simulink library "tqd"  (R2021b)
settings: Solver=VariableStepAuto  StartTime=0.0  StopTime=10.0  RelTol=1e-3
undefined symbols (not defined in the file or in its folder): ATQD_APSDecReq_X_kph, ATQD_APSDecReq_Y_mps2, ATQD_APSDecReqCMD_X_kph, ATQD_APSDecReqTs_X_pct, ATQD_APSDecTimeGain_X_Deg, ATQD_APSDecTimeGain_Y_s, ATQD_APSReqLowSpd_X_Deg, ATQD_AutoHoldReleaseBPS_X_Deg, ATQD_AWDLoadTrqnsGain_X_kg, ATQD_AWDLoadTrqnsGain_Y_pct, ATQD_BOSEnBPSPosn_X_kph, ATQD_BOSMap_X_rpm, ATQD_BOSMap_Y_pct, ATQD_CreepBaseTqD_X_kph, ATQD_CreepBaseTqD_Y_Deg, ATQD_CreepBaseTqR_X_kph, ATQD_CreepBaseTqR_Y_Deg, ATQD_CreepBPSDisPosn_X_Deg, ATQD_CreepBPSDisPosnR_X_Deg, ATQD_CreepBPSEnPosn_X_Deg, ATQD_CreepBPSEnPosnR_X_Deg, ATQD_CreepDeltaTq_X_kph, ATQD_CreepIterm_X_kph, ATQD_CreepIterm_Y_kph, ATQD_CreepItermMaxLimit_X_pct, ATQD_CreepPreloadTime_X_kph, ATQD_CreepPreloadTq_X_kph, ATQD_CreepPreloadTq_Y_s, ATQD_CreepProtTq_X_Deg, ATQD_CreepPterm_X_kph, ATQD_ECOTqMapD_X_rpm, ATQD_ECOTqMapD_Y_pct, ATQD_EOPDTqMapDCon_X_rpm, ATQD_EOPDTqMapDCon_Y_Deg, ATQD_EstInitVehWeight_X_c, ATQD_LHMRollGenMapD_X_rpm, ATQD_LHMRollGenMapD_Y_rpm, ATQD_LHMTqMapD_X_rpm, ATQD_LHMTqMapD_Y_pct, ATQD_NL1TqMapD_X_rpm, ATQD_NL1TqMapD_Y_pct, ATQD_NOPDTqMapDCon_X_rpm, ATQD_NOPDTqMapDCon_Y_Deg, ATQD_NRMRrEDUSpRat_X_rpm, ATQD_NRMRrEDUSpRat_Y_Nm, ATQD_OPDHoldDownRelDelay_X_Deg, ATQD_OPDHoldEnSpd_X_Deg, ATQD_OPDHoldRelDetTime_X_Deg, ATQD_OPDHoldReleaseTq_X_Deg, ATQD_OrigPedTqLowLim_X_Deg, ATQD_OrigPedTqLowLim_Y_pct, ATQD_PedalMapClimbUpLim_X_rpm, ATQD_PedalMapClimbUpLim_Y_Deg, ATQD_PreLoadTq_X_s, ATQD_RollGenMapEL1_X_rpm, ATQD_RollGenMapEL1_Y_rpm, ATQD_SL1TqMapD_X_rpm, ATQD_SL1TqMapD_Y_pct, ATQD_SlideRegenTqGain_X_Gps, ATQD_SlideRegenTqGain_Y_pct ... (+444)
libraries: hcu_lib x70, simulink x61, tqr x1
(part 11 of 14)

== system tqd/TQD/TorqueDemand/TorqueModule/OPD Hold/Release Condition ==
  VVMC_EstSlope_Deg : Inport
  VTQD_VehActSpd_kph : Inport  Port=2
  VTQR_NoABSFEDUWhlTqReq_Nm : Inport  Port=3
  VTQR_NoABSREDUWhlTqReq_Nm : Inport  Port=4
  VTQD_ActBPSPosn_pct : Inport  Port=5
  task_time_s : Inport  Port=6
  VTQD_APSReqTimer_s : Inport  Port=7
  VTQD_LowIdleAccPedal_flg : Inport  Port=8
  VTQD_OPDHoldRgnOn2Off_flg : Inport  Port=9
  VTQD_ActAPSPosn_pct : Inport  Port=10
  VTQD_FrOPDHoldRelTqGain_Nm : Inport  Port=11
  VTQD_RrOPDHoldRelTqGain_Nm : Inport  Port=12
  AND : Logic  Inputs=3  AllPortsSameDT=off  OutDataTypeStr=boolean
  AND1 : Logic  AllPortsSameDT=off  OutDataTypeStr=boolean
  AND2 : Logic  AllPortsSameDT=off  OutDataTypeStr=boolean
  AND3 : Logic  AllPortsSameDT=off  OutDataTypeStr=boolean
  Add : Sum
  Add1 : Sum  Inputs=+-+
  Add6 : Sum
  Add7 : Sum
  Constant1 : Constant  Value=KTQD_APSRelDisTqDev_Nm
  Constant{5,10,23,30} (4 alike) : Constant  Value=ZERO_FLOAT
  Constant2 : Constant  Value=KTQD_OPDHoldDownEnTime_s
  Constant36 : Constant  Value=KTQD_OPDHoldRelDetSpd_kph
  Constant4 : Constant  Value=KTQD_OPDHoldRelTqGain_Nm
  Constant6 : Constant  Value=KTQD_OPDHoldDetRevSpd_kph
  Constant7 : Constant  Value=KTQD_OPDHoldLiftRevSpd_kph
  Constant8 : Constant  Value=KTQD_APSDecReqMaxTime_s
  Constant9 : Constant  Value=KTQD_OPDHoldRelTqGain_Nm
  Delay{,1..3} (4 alike) : Delay  DelayLength=1
  DelayEnable : hcu_lib/Basic_Blocks/DelayEnable
  DelayEnable1 : hcu_lib/Basic_Blocks/DelayEnable
  Detect Increase : simulink/Logic and Bit Operations/Detect Increase  vinit=0.0  OutDataTypeStr=boolean
  Detect Increase1 : simulink/Logic and Bit Operations/Detect Increase  vinit=0.0  OutDataTypeStr=boolean
  Detect Increase2 : simulink/Logic and Bit Operations/Detect Increase  vinit=0.0  OutDataTypeStr=boolean
  MTQD_AutoHoldReleaseBPS_Y_pct : Lookup_n-D  NumberOfTableDimensions=1  BreakpointsForDimension1=ATQD_AutoHoldReleaseBPS_X_Deg  Table=MTQD_AutoHoldReleaseBPS_Y_pct  InternalRulePriority=Speed  RndMeth=Simplest  InputSameDT=on
  MTQD_OPDHoldDownRelDelay_Y_s : Lookup_n-D  NumberOfTableDimensions=1  BreakpointsForDimension1=ATQD_OPDHoldDownRelDelay_X_Deg  Table=MTQD_OPDHoldDownRelDelay_Y_s  InternalRulePriority=Speed  RndMeth=Simplest  InputSameDT=on
  MTQD_OPDHoldRelDetTime_Y_s : Lookup_n-D  NumberOfTableDimensions=1  BreakpointsForDimension1=ATQD_OPDHoldRelDetTime_X_Deg  Table=MTQD_OPDHoldRelDetTime_Y_s  InternalRulePriority=Speed  RndMeth=Simplest  InputSameDT=on
  MTQD_OPDHoldReleaseTq_Y_Nm{,1..3} (4 alike) : Lookup_n-D  NumberOfTableDimensions=1  BreakpointsForDimension1=ATQD_OPDHoldReleaseTq_X_Deg  Table=MTQD_OPDHoldReleaseTq_Y_Nm  InternalRulePriority=Speed  RndMeth=Simplest  InputSameDT=on
  Max : MinMax  Function=max  Inputs=2
  Max1 : MinMax  Function=max  Inputs=2
  Max2 : MinMax  Function=max  Inputs=2
  NOT{,1..5} (6 alike) : Logic  Operator=NOT  AllPortsSameDT=off  OutDataTypeStr=boolean
  OR : Logic  Operator=OR  AllPortsSameDT=off  OutDataTypeStr=boolean
  OR1 : Logic  Operator=OR  AllPortsSameDT=off  OutDataTypeStr=boolean
  OR2 : Logic  Operator=OR  AllPortsSameDT=off  OutDataTypeStr=boolean
  OR3 : Logic  Operator=OR  Inputs=3  AllPortsSameDT=off  OutDataTypeStr=boolean
  Relational Operator : RelationalOperator  Operator=>  OutDataTypeStr=boolean  RndMeth=Simplest
  Relational Operator1 : RelationalOperator  Operator=<=  OutDataTypeStr=boolean  RndMeth=Simplest
  Relational Operator3 : RelationalOperator  Operator=<=  OutDataTypeStr=boolean  RndMeth=Simplest
  Relational Operator4 : RelationalOperator  OutDataTypeStr=boolean  RndMeth=Simplest
  Relational Operator5 : RelationalOperator  Operator=<  OutDataTypeStr=boolean  RndMeth=Simplest
  Relational Operator6 : RelationalOperator  Operator=>  OutDataTypeStr=boolean  RndMeth=Simplest
  Relational Operator7 : RelationalOperator  OutDataTypeStr=boolean  RndMeth=Simplest
  Relational Operator9 : RelationalOperator  OutDataTypeStr=boolean  RndMeth=Simplest
  Relay : Relay  OnSwitchValue=KTQD_OPDHoldGradeUp_Deg  OffSwitchValue=KTQD_OPDHoldGradeDown_Deg  OutDataTypeStr=boolean
  Relay1 : Relay  OnSwitchValue=KTQD_OPDHoldGradeUp_Deg  OffSwitchValue=KTQD_OPDHoldGradeDown_Deg  OutDataTypeStr=boolean
  SR_Latch : hcu_lib/Basic_Blocks/SR_Latch
  SR_Latch1 : hcu_lib/Basic_Blocks/SR_Latch
  Switch{,1..6} (7 alike) : Switch  Criteria=u2 > Threshold
  Terminator : Terminator
  VTQD_AutoHoldRelease_flg : Outport
  VTQD_OPDHoldEnRel_flg : Outport  Port=2
  VTQD_OPDHoldActRelTq_Nm : Outport  Port=3
  wires:
  VVMC_EstSlope_Deg/1 -> [VVMC_EstSlope_Deg]
  VTQD_VehActSpd_kph/1 -> [VTQD_VehActSpd_kph]
  VTQR_NoABSFEDUWhlTqReq_Nm/1 -> [VTQR_NoABSFEDUWhlTqReq_Nm]
  VTQR_NoABSREDUWhlTqReq_Nm/1 -> [VTQR_NoABSREDUWhlTqReq_Nm]
  VTQD_ActBPSPosn_pct/1 -> [VTQD_ActBPSPosn_pct]
  task_time_s/1 -> [task_time_s]
  [VTQD_AutoHoldRelease_flg] -> VTQD_AutoHoldRelease_flg/1
  [VTQD_OPDHoldEnRel_flg] -> VTQD_OPDHoldEnRel_flg/1
  VTQD_APSReqTimer_s/1 -> [VTQD_APSReqTimer_s]
  VTQD_LowIdleAccPedal_flg/1 -> [VTQD_LowIdleAccPedal_flg]
  VTQD_OPDHoldRgnOn2Off_flg/1 -> [VTQD_OPDHoldRgnOn2Off_flg]
  VTQD_ActAPSPosn_pct/1 -> Terminator/1
  VTQD_RrOPDHoldRelTqGain_Nm/1 -> [VTQD_RrOPDHoldRelTqGain_Nm]
  VTQD_FrOPDHoldRelTqGain_Nm/1 -> [VTQD_FrOPDHoldRelTqGain_Nm]
  SR_Latch/1 -> DelayEnable/1  "VTQD_OPDHoldEnRelLatch_flg"
  Detect Increase2/1 -> OR2/1
  Detect Increase1/1 -> SR_Latch1/1
  DelayEnable1/1 -> Switch1/1
  SR_Latch1/1 -> [VTQD_OPDHoldRelReverse_flg]  "VTQD_OPDHoldRelReverse_flg"
  MTQD_OPDHoldDownRelDelay_Y_s/1 -> [VTQD_OPDHoldDownRelDelay_s]  "VTQD_OPDHoldDownRelDelay_s"
  Constant4/1 -> Switch2/1
  [VVMC_EstSlope_Deg] -> MTQD_OPDHoldDownRelDelay_Y_s/1
  [task_time_s] -> DelayEnable1/3
  [VTQD_LowIdleAccPedal_flg] -> NOT2/1
  Constant30/1 -> Switch5/1
  NOT/1 -> AND/2
  [VVMC_EstSlope_Deg] -> Relay1/1
  Relay1/1 -> NOT3/1
  Constant2/1 -> Relational Operator1/2
  OR1/1 -> AND/3
  Switch1/1 -> Switch/3
  AND2/1 -> Switch1/3
  [VTQD_LowIdleAccPedal_flg] -> NOT1/1
  [VTQD_OPDHoldRgnOn2Off_flg] -> Switch/2
  Relational Operator/1 -> OR1/1
  Relational Operator1/1 -> AND/1
  [VTQD_OPDHoldRelDetTime_s] -> DelayEnable/2
  AND/1 -> OR/1
  [VVMC_EstSlope_Deg] -> Relay/1
  [VTQR_NoABSFEDUWhlTqReq_Nm] -> Add6/1
  [VTQR_NoABSREDUWhlTqReq_Nm] -> Add6/2
  [task_time_s] -> DelayEnable/3
  [VTQR_NoABSFEDUWhlTqReq_Nm] -> Add7/1
  [VTQD_ActBPSPosn_pct] -> Relational Operator/1
  Add1/1 -> Max1/1
  [VVMC_EstSlope_Deg] -> MTQD_OPDHoldReleaseTq_Y_Nm/1
  DelayEnable/1 -> [VTQD_OPDHoldEnRel_flg]  "VTQD_OPDHoldEnRel_flg"
  [VTQR_NoABSREDUWhlTqReq_Nm] -> Add7/2
  Max1/1 -> Relational Operator5/2
  [VTQD_VehActSpd_kph] -> Relational Operator9/1
  Relational Operator9/1 -> Switch5/2
  [VVMC_EstSlope_Deg] -> MTQD_AutoHoldReleaseBPS_Y_pct/1
  [VVMC_EstSlope_Deg] -> MTQD_OPDHoldRelDetTime_Y_s/1
  Switch5/1 -> [VTQD_OPDHoldRelDetTime_s]  "VTQD_OPDHoldRelDetTime_s"
  MTQD_AutoHoldReleaseBPS_Y_pct/1 -> Relational Operator/2  "VTQD_AutoHoldReleaseAPS_pct"
  OR/1 -> [VTQD_AutoHoldRelease_flg]  "VTQD_AutoHoldRelease_flg"
  MTQD_OPDHoldReleaseTq_Y_Nm/1 -> Switch6/3
  Relational Operator3/1 -> Detect Increase1/1
  [VTQD_OPDHoldDownRelDelay_s] -> DelayEnable1/2
  Delay3/1 -> Max2/1
  Max2/1 -> Switch6/1
  Constant6/1 -> Relational Operator3/2
  Detect Increase/1 -> OR3/1
  Add7/1 -> Relational Operator5/1  "VTQD_OPDHoldDisRelTq_Nm"
  Switch6/1 -> Add/2, Delay3/1  "VTQD_OPDHoldReleaseTq_Nm"
  [VVMC_EstSlope_Deg] -> MTQD_OPDHoldReleaseTq_Y_Nm3/1
  [VTQD_APSReqTimer_s] -> Delay/1
  NOT3/1 -> Switch1/2
  [VTQD_OPDHoldRelReverse_flg] -> Detect Increase2/1
  [VTQD_OPDHoldRelReverse_flg] -> Switch6/2
  Constant23/1 -> Max1/2
  [VTQD_LowIdleAccPedal_flg] -> NOT4/1
  MTQD_OPDHoldRelDetTime_Y_s/1 -> Switch5/3
  [VTQD_OPDHoldRelReverse_flg] -> Switch3/2
  Relational Operator4/1 -> SR_Latch/1  "VTQD_OPDHoldEnRelease_flg"
  Switch2/1 -> Add/1
  NOT5/1 -> AND2/2
  MTQD_OPDHoldReleaseTq_Y_Nm1/1 -> Switch4/3
  Relay/1 -> NOT/1
  Add/1 -> [VTQD_OPDHoldActRelTq_Nm], Relational Operator4/2  "VTQD_OPDHoldActRelTq_Nm"
  [VTQD_OPDHoldRelReverse_flg] -> Switch4/2
  Delay/1 -> Relational Operator1/1
  Constant8/1 -> Relational Operator7/2
  OR2/1 -> SR_Latch/2
  [VTQD_VehActSpd_kph] -> Relational Operator3/1
  Delay2/1 -> Max/1
  [VTQD_OPDHoldEnRel_flg] -> AND1/2
  AND1/1 -> Switch/1
  [VTQD_LowIdleAccPedal_flg] -> AND3/1
  [VTQD_LowIdleAccPedal_flg] -> NOT5/1
  Constant36/1 -> Relational Operator9/2
  NOT4/1 -> DelayEnable1/1
  [VTQD_APSReqTimer_s] -> Delay1/1
  Constant10/1 -> Switch3/3
  MTQD_OPDHoldReleaseTq_Y_Nm2/1 -> Max/2
  [VTQD_LowIdleAccPedal_flg] -> Detect Increase/1
  Add6/1 -> Relational Operator4/1  "VTQD_OPDHoldEnRelTq_flg"
  [VTQD_OPDHoldRelReverse_flg] -> Switch2/2
  Switch3/1 -> Add1/1
  [VVMC_EstSlope_Deg] -> MTQD_OPDHoldReleaseTq_Y_Nm1/1
  Relational Operator5/1 -> OR2/2  "VTQD_OPDHoldDisRelease_flg"
  MTQD_OPDHoldReleaseTq_Y_Nm3/1 -> Max2/2
  Delay1/1 -> Relational Operator7/1
  Relational Operator7/1 -> AND3/2
  Constant7/1 -> Relational Operator6/2
  Switch4/1 -> Delay2/1, Add1/3
  Constant5/1 -> Switch2/3
  AND3/1 -> OR3/3
  Constant9/1 -> Switch3/1
  Switch/1 -> OR/2
  NOT2/1 -> AND1/1
  [VTQD_VehActSpd_kph] -> Relational Operator6/1
  [VTQD_OPDHoldEnRel_flg] -> AND2/1
  Constant1/1 -> Add1/2
  NOT1/1 -> OR1/2
  Relational Operator6/1 -> OR3/2
  Max/1 -> Switch4/1
  [VVMC_EstSlope_Deg] -> MTQD_OPDHoldReleaseTq_Y_Nm2/1
  OR3/1 -> SR_Latch1/2
  [VTQD_OPDHoldActRelTq_Nm] -> VTQD_OPDHoldActRelTq_Nm/1

== system tqd/TQD/TorqueDemand/TorqueModule/OPD Hold/System Status ==
  VTQD_GearActualPosn_enum : Inport
  VINP_EPBSta_enum : Inport  Port=2
  VTQD_RegenMode_enum : Inport  Port=3
  VTQD_AutiHoldRelease_flg : Inport  Port=4
  VTQD_AntiBlockRrActDisTime_s : Inport  Port=5
  VTQD_RrAntiBlockAactive_flg : Inport  Port=6
  VTQD_ActBPSPosn_pct : Inport  Port=7
  VTQD_AntiBlockFrActDisTime_s : Inport  Port=8
  VTQD_FrAntiBlockAactive_flg : Inport  Port=9
  VVMC_ADASActive_flg : Inport  Port=10
  VPMM_PwrSta_enum : Inport  Port=11
  VVMC_CruzActive_flg : Inport  Port=12
  VTQD_VehActSpd_kph : Inport  Port=13
  AND2 : Logic  Inputs=6  AllPortsSameDT=off  OutDataTypeStr=boolean
  AND5 : Logic  AllPortsSameDT=off  OutDataTypeStr=boolean
  AND6 : Logic  AllPortsSameDT=off  OutDataTypeStr=boolean
  Constant1 : Constant  Value=2  OutDataTypeStr=uint8
  Constant2 : Constant  Value=0  OutDataTypeStr=uint8
  Constant3 : Constant  Value=ENUM_EPBSTA_APPLIED
  Constant4 : Constant  Value=ENUM_GEARACTUALPOSN_P
  Constant40 : Constant  Value=ENUM_REGENLEVEL_OPD
  Constant44 : Constant  Value=ENUM_REGENLEVEL_OPD
  Constant45 : Constant  Value=ENUM_POWERSTA_READY
  Constant5 : Constant  Value=ENUM_GEARACTUALPOSN_D
  Constant6 : Constant  Value=KTQD_AutoHoldEnSpd_kph
  Constant7 : Constant  Value=ENUM_EPBSTA_APPLIED
  Delay : Delay  DelayLength=1
  Equal{1..2,8,11,30} (5 alike) : RelationalOperator  Operator===  OutDataTypeStr=boolean  RndMeth=Simplest
  Equal10 : RelationalOperator  Operator=~=  OutDataTypeStr=boolean  RndMeth=Simplest
  Equal3 : RelationalOperator  Operator=~=  OutDataTypeStr=boolean  RndMeth=Simplest
  GreaterThan3 : RelationalOperator  Operator=>  OutDataTypeStr=boolean  RndMeth=Simplest
  NOT3 : Logic  Operator=NOT  AllPortsSameDT=off  OutDataTypeStr=boolean
  NOT4 : Logic  Operator=NOT  AllPortsSameDT=off  OutDataTypeStr=boolean
  OR1 : Logic  Operator=OR  AllPortsSameDT=off  OutDataTypeStr=boolean
  OR5 : Logic  Operator=OR  AllPortsSameDT=off  OutDataTypeStr=boolean
  Relational Operator3 : RelationalOperator  Operator=<=  OutDataTypeStr=boolean  RndMeth=Simplest
  SR_Latch3 : hcu_lib/Basic_Blocks/SR_Latch
  Switch : Switch  Criteria=u2 > Threshold
  Unit Delay1 : UnitDelay  SampleTime=-1  HasFrameUpgradeWarning=on
  VTQD_APSStaSys_enum : Outport
  VTQD_OPDHoldDelayForP_flg : Outport  Port=2
  VTQD_OPDHoldRgnOn2Off_flg : Outport  Port=3
  wires:
  Constant6/1 -> Relational Operator3/2
  [VVMC_CruzActive_flg] -> NOT4/1
  NOT4/1 -> AND2/4
  Relational Operator3/1 -> AND2/5
  OR1/1 -> AND2/3
  Switch/1 -> [VTQD_APSStaSys_enum]  "VTQD_APSStaSys_enum"
  [VTQD_VehActSpd_kph] -> Relational Operator3/1
  Equal2/1 -> OR1/1
  Constant2/1 -> Switch/3
  AND2/1 -> Switch/2
  Constant1/1 -> Switch/1
  [VTQD_GearActualPosn_enum] -> Equal2/1
  [VTQD_GearActualPosn_enum] -> Equal1/1
  Equal1/1 -> AND5/1
  AND5/1 -> [VTQD_OPDHoldDelayForP_flg]  "VTQD_OPDHoldDelayForP_flg"
  Equal10/1 -> AND5/2
  [VTQD_RegenMode_enum] -> Equal8/1
  OR5/1 -> [VTQD_AntiBlockEnOPDHold_flg]  "VTQD_AntiBlockEnOPDHold_flg"
  Equal8/1 -> OR5/2
  Constant40/1 -> Equal8/2
  Equal11/1 -> GreaterThan3/2, Unit Delay1/1
  SR_Latch3/1 -> [VTQD_OPDHoldRgnOn2Off_flg]  "VTQD_OPDHoldRgnOn2Off_flg"
  GreaterThan3/1 -> AND6/2
  Constant45/1 -> Equal30/2
  AND6/1 -> SR_Latch3/1
  [VPMM_PwrSta_enum] -> Equal30/1
  Equal30/1 -> AND6/1
  Unit Delay1/1 -> GreaterThan3/1
  [VTQD_AutiHoldRelease_flg] -> Delay/1
  Constant44/1 -> Equal11/2
  [VTQD_RegenMode_enum] -> Equal11/1
  Constant3/1 -> Equal10/2
  [VINP_EPBSta_enum] -> Equal10/1
  Constant4/1 -> Equal1/2
  Constant5/1 -> Equal2/2
  [VVMC_ADASActive_flg] -> NOT3/1
  NOT3/1 -> AND2/1
  [VTQD_AntiBlockEnOPDHold_flg] -> AND2/2
  [VTQD_OPDHoldRgnOn2Off_flg] -> OR5/1
  VTQD_GearActualPosn_enum/1 -> [VTQD_GearActualPosn_enum]
  VINP_EPBSta_enum/1 -> [VINP_EPBSta_enum]
  VTQD_RegenMode_enum/1 -> [VTQD_RegenMode_enum]
  VTQD_AutiHoldRelease_flg/1 -> [VTQD_AutiHoldRelease_flg]
  VTQD_AntiBlockRrActDisTime_s/1 -> [VTQD_AntiBlockRrActDisTime_s]
  VTQD_RrAntiBlockAactive_flg/1 -> [VTQD_RrAntiBlockAactive_flg]
  VTQD_ActBPSPosn_pct/1 -> [VTQD_ActBPSPosn_pct]
  VTQD_AntiBlockFrActDisTime_s/1 -> [VTQD_AntiBlockFrActDisTime_s]
  VTQD_FrAntiBlockAactive_flg/1 -> [VTQD_FrAntiBlockAactive_flg]
  VVMC_ADASActive_flg/1 -> [VVMC_ADASActive_flg]
  VPMM_PwrSta_enum/1 -> [VPMM_PwrSta_enum]
  [VTQD_OPDHoldDelayForP_flg] -> OR1/2
  VVMC_CruzActive_flg/1 -> [VVMC_CruzActive_flg]
  VTQD_VehActSpd_kph/1 -> [VTQD_VehActSpd_kph]
  [VTQD_APSStaSys_enum] -> VTQD_APSStaSys_enum/1
  [VTQD_OPDHoldDelayForP_flg] -> VTQD_OPDHoldDelayForP_flg/1
  [VTQD_OPDHoldRgnOn2Off_flg] -> VTQD_OPDHoldRgnOn2Off_flg/1
  Constant7/1 -> Equal3/2
  [VINP_EPBSta_enum] -> Equal3/1
  Equal3/1 -> AND2/6
  Delay/1 -> SR_Latch3/2

== system tqd/TQD/TorqueDemand/TorqueModule/TqCoordination/Coordinate_ADAS ==
  VVMC_ADASWhlTqReq_Nm : Inport
  VTQD_PreLoadHold_flg : Inport  Port=2
  VTQD_DriverWhlTqDem_Nm : Inport  Port=3
  Action Port : ActionPort
  Constant9 : Constant  Value=ENUM_TQSOURCE_ADAS
  Switch : Switch  Criteria=u2 > Threshold
  VTQD_ADASWhlTqReq_Nm : Outport
  VTQD_TqSourceADAS_enum : Outport  Port=2
  wires:
  VTQD_DriverWhlTqDem_Nm/1 -> Switch/1
  Switch/1 -> VTQD_ADASWhlTqReq_Nm/1
  VTQD_PreLoadHold_flg/1 -> Switch/2
  Constant9/1 -> VTQD_TqSourceADAS_enum/1
  VVMC_ADASWhlTqReq_Nm/1 -> Switch/3

== system tqd/TQD/TorqueDemand/TorqueModule/TqCoordination/Coordinate_ADASForceIdle ==
  Action Port : ActionPort
  Constant : Constant  Value=ZERO_FLOAT
  Constant8 : Constant  Value=ENUM_TQSOURCE_ADASFORCEIDLE
  VTQD_ADASForceIdleReq_Nm : Outport
  VTQD_ADASForceIdle_enum : Outport  Port=2
  wires:
  Constant8/1 -> VTQD_ADASForceIdle_enum/1
  Constant/1 -> VTQD_ADASForceIdleReq_Nm/1

== system tqd/TQD/TorqueDemand/TorqueModule/TqCoordination/Coordinate_APS ==
  VTQD_DriverWhlTqDem_Nm : Inport
  Action Port : ActionPort
  Constant9 : Constant  Value=ENUM_TQSOURCE_APS
  VTQD_APSWhlTqReq_Nm : Outport
  VTQD_TqSourceAPS_enum : Outport  Port=2
  wires:
  Constant9/1 -> VTQD_TqSourceAPS_enum/1
  VTQD_DriverWhlTqDem_Nm/1 -> VTQD_APSWhlTqReq_Nm/1

== system tqd/TQD/TorqueDemand/TorqueModule/TqCoordination/Coordinate_Cruise ==
  VVMC_CruzWhlTqReq_Nm : Inport
  Action Port : ActionPort
  Constant9 : Constant  Value=ENUM_TQSOURCE_CC
  VTQD_CruzWhlTqReq_Nm : Outport
  VTQD_TqSourceCruz_enum : Outport  Port=2
  wires:
  Constant9/1 -> VTQD_TqSourceCruz_enum/1
  VVMC_CruzWhlTqReq_Nm/1 -> VTQD_CruzWhlTqReq_Nm/1

== system tqd/TQD/TorqueDemand/TorqueModule/TqCoordination/Coordinate_DirverPedal ==
  VTQD_DriverWhlTqDem_Nm : Inport
  Action Port : ActionPort
  Constant9 : Constant  Value=ENUM_TQSOURCE_INTERNAL
  VTQD_DriverWhlTqReq_Nm : Outport
  VTQD_TqSourceInternal_enum : Outport  Port=2
  wires:
  VTQD_DriverWhlTqDem_Nm/1 -> VTQD_DriverWhlTqReq_Nm/1
  Constant9/1 -> VTQD_TqSourceInternal_enum/1

== system tqd/TQD/TorqueDemand/TorqueModule/TqCoordination/Coordinate_MSA ==
  VVMC_MSAWhlTqReq_Nm : Inport
  Action Port : ActionPort
  Constant9 : Constant  Value=ENUM_TQSOURCE_MSA
  VTQD_MSAWhlTqReq_Nm : Outport
  VTQD_TqSourceMSA_enum : Outport  Port=2
  wires:
  Constant9/1 -> VTQD_TqSourceMSA_enum/1
  VVMC_MSAWhlTqReq_Nm/1 -> VTQD_MSAWhlTqReq_Nm/1

== system tqd/TQD/TorqueDemand/TorqueModule/TqCoordination/Coordinate_NoSuitbleGear_flg ==
  Action Port : ActionPort
  Constant5 : Constant  Value=KTQD_DriverTqDemN_Nm
  Constant8 : Constant  Value=ENUM_TQSOURCE_INVALID
  VTQD_GearNoSuitReq_Nm : Outport
  VTQD_TqSourceGearNoSuit_enum : Outport  Port=2
  wires:
  Constant5/1 -> VTQD_GearNoSuitReq_Nm/1
  Constant8/1 -> VTQD_TqSourceGearNoSuit_enum/1

== system tqd/TQD/TorqueDemand/TorqueModule/TqDistribution/AWD_Ratio ==
  note: initia:2000kg
  VTQD_DriverWhlTqDem_Nm : Inport
  VTQD_RrShaftSpd_rpm : Inport  Port=2
  VTQD_EVDriveMode_enum : Inport  Port=3
  VTQD_LimpHomeAct_flg : Inport  Port=4
  VVMC_APSActive_flg : Inport  Port=5
  VTQD_CreepPrLoadEnable_flg : Inport  Port=6
  VTQD_EstVehWeightResult_kg : Inport  Port=7
  VVMC_ActLRSlideRate_pct : Inport  Port=8
  VVMC_ActRRSlideRate_pct : Inport  Port=9
  VVMC_RearTqRatio_rat : Inport  Port=10
  Action Port : ActionPort
  AND : Logic  AllPortsSameDT=off  OutDataTypeStr=boolean
  Abs : Abs
  Abs1 : Abs
  Constant : Constant  Value=ONE_FLOAT
  Constant1 : Constant  Value=ONE_FLOAT
  Constant10 : Constant  Value=KTQD_AWDRrRatio_rat_ovrdflg  VectorParams1D=off  SampleTime=-1
  Constant11 : Constant  Value=KTQD_AWDRrRatio_rat_ovrdval  VectorParams1D=off  SampleTime=-1
  Constant12 : Constant  Value=KTQD_DrvSelPwrTrainSW_flg  VectorParams1D=off  SampleTime=-1
  Constant13 : Constant  Value=KTQD_AWDWhlTqRatioSW_flg
  Constant14 : Constant  Value=KTQD_WhlRatioDisCreep_flg
  Constant2 : Constant  Value=ENUM_DRIVEMODE_ECO
  Constant3 : Constant  Value=ENUM_DRIVETRAIN_FWD  VectorParams1D=off  SampleTime=-1
  Constant4 : Constant  Value=ENUM_DRIVETRAIN_AWD  VectorParams1D=off  SampleTime=-1
  Constant5 : Constant  Value=ENUM_DRIVEMODE_SPORT
  Constant6 : Constant  Value=ZERO_FLOAT
  Constant7 : Constant  Value=ONE_FLOAT
  Constant8 : Constant  Value=KTQD_AWDFrRatio_rat_ovrdflg  VectorParams1D=off  SampleTime=-1
  Constant9 : Constant  Value=KTQD_AWDFrRatio_rat_ovrdval  VectorParams1D=off  SampleTime=-1
  Equal : RelationalOperator  Operator===  OutDataTypeStr=boolean  RndMeth=Simplest
  Equal1 : RelationalOperator  Operator=~=  OutDataTypeStr=boolean  RndMeth=Simplest
  Equal2 : RelationalOperator  Operator===  OutDataTypeStr=boolean  RndMeth=Simplest
  Equal3 : RelationalOperator  Operator===  OutDataTypeStr=boolean  RndMeth=Simplest
  Ground : Ground
  LiuzgSwitch{1..5,13} (6 alike) : Switch  Criteria=u2 ~= 0
      settings: AttributesFormatString=<%<Criteria>>
  MTQD_AWDLoadTrqnsGain_Z_c : Lookup_n-D  BreakpointsForDimension1=ATQD_AWDLoadTrqnsGain_Y_pct  BreakpointsForDimension2=ATQD_AWDLoadTrqnsGain_X_kg  Table=MTQD_AWDLoadTrqnsGain_Z_c  ExtrapMethod=Clip  InternalRulePriority=Speed  RndMeth=Simplest  InputSameDT=on
      settings: InputPortMap=u0,u1
  MTQD_ECORrEDUSpRat_Z_rat : Lookup_n-D  BreakpointsForDimension1=ATQD_NRMRrEDUSpRat_Y_Nm  BreakpointsForDimension2=ATQD_NRMRrEDUSpRat_X_rpm  Table=MTQD_ECORrEDUSpRat_Z_rat  ExtrapMethod=Clip  InternalRulePriority=Speed  RndMeth=Simplest  InputSameDT=on
      settings: InputPortMap=u0,u1
  "MTQD_NRMRrEDUSpRat_Z_rat  " : Lookup_n-D  BreakpointsForDimension1=ATQD_NRMRrEDUSpRat_Y_Nm  BreakpointsForDimension2=ATQD_NRMRrEDUSpRat_X_rpm  Table=MTQD_NRMRrEDUSpRat_Z_rat  ExtrapMethod=Clip  InternalRulePriority=Speed  RndMeth=Simplest  InputSameDT=on
      settings: InputPortMap=u0,u1
  "MTQD_SPORTRrEDUSpRat_Z_rat " : Lookup_n-D  BreakpointsForDimension1=ATQD_NRMRrEDUSpRat_Y_Nm  BreakpointsForDimension2=ATQD_NRMRrEDUSpRat_X_rpm  Table=MTQD_SPORTRrEDUSpRat_Z_rat  ExtrapMethod=Clip  InternalRulePriority=Speed  RndMeth=Simplest  InputSameDT=on
      settings: InputPortMap=u0,u1
  Max : MinMax  Function=max  Inputs=2
  NOT : Logic  Operator=NOT  AllPortsSameDT=off  OutDataTypeStr=boolean
  OR : Logic  Operator=OR  AllPortsSameDT=off  OutDataTypeStr=boolean
  OR1 : Logic  AllPortsSameDT=off  OutDataTypeStr=boolean
  Product : Product
  Saturation : Saturate  UpperLimit=KTQD_RrEDUTqDistrictMax_gain  LowerLimit=KTQD_RrEDUTqDistrictMin_gain
      settings: AttributesFormatString=|
      | <%<UpperLimit>>
      | <%<LowerLimit>>
  Subtract : Sum  Inputs=+-
  Switch : Switch  Criteria=u2 > Threshold
  Switch1 : Switch  Criteria=u2 > Threshold
  Switch2 : Switch  Criteria=u2 > Threshold
  VTQD_FrRatio_AWD : Outport
  VTQD_RrRatio_AWD : Outport  Port=2
  wires:
  Constant/1 -> Subtract/1
  Saturation/1 -> Switch1/3, Subtract/2
  VTQD_EVDriveMode_enum/1 -> [VTQD_EVDriveMode_enum]
  VTQD_DriverWhlTqDem_Nm/1 -> [VTQD_DriverWhlTqDem_Nm]
  VTQD_RrShaftSpd_rpm/1 -> [VTQD_RrShaftSpd_rpm]
  [VTQD_DriverWhlTqDem_Nm] -> "MTQD_NRMRrEDUSpRat_Z_rat  "/1
  [VTQD_RrShaftSpd_rpm] -> "MTQD_NRMRrEDUSpRat_Z_rat  "/2
  VTQD_LimpHomeAct_flg/1 -> [VTQD_LimpHomeAct_flg]
  [VTQD_LimpHomeAct_flg] -> LiuzgSwitch13/2
  Equal/1 -> LiuzgSwitch1/2
  "MTQD_SPORTRrEDUSpRat_Z_rat "/1 -> LiuzgSwitch1/1
  [VTQD_EVDriveMode_enum] -> Equal/1
  Constant5/1 -> Equal/2
  [VTQD_DriverWhlTqDem_Nm] -> "MTQD_SPORTRrEDUSpRat_Z_rat "/1
  [VTQD_RrShaftSpd_rpm] -> "MTQD_SPORTRrEDUSpRat_Z_rat "/2
  "MTQD_NRMRrEDUSpRat_Z_rat  "/1 -> LiuzgSwitch1/3, LiuzgSwitch13/1
  [VTQD_RrShaftSpd_rpm] -> MTQD_ECORrEDUSpRat_Z_rat/2
  [VTQD_DriverWhlTqDem_Nm] -> MTQD_ECORrEDUSpRat_Z_rat/1
  Constant2/1 -> Equal2/2
  [VTQD_EVDriveMode_enum] -> Equal2/1
  MTQD_ECORrEDUSpRat_Z_rat/1 -> LiuzgSwitch3/1
  Equal2/1 -> LiuzgSwitch3/2
  LiuzgSwitch3/1 -> LiuzgSwitch13/3
  LiuzgSwitch1/1 -> LiuzgSwitch3/3
  OR/1 -> OR1/1
  [VTQD_CreepPrLoadEnable_flg] -> OR/2
  Constant1/1 -> LiuzgSwitch2/1
  [VVMC_APSActive_flg] -> OR/1
  VVMC_APSActive_flg/1 -> [VVMC_APSActive_flg]
  VTQD_CreepPrLoadEnable_flg/1 -> [VTQD_CreepPrLoadEnable_flg]
  Product/1 -> Switch2/3
  LiuzgSwitch13/1 -> Product/1
  MTQD_AWDLoadTrqnsGain_Z_c/1 -> [VTQD_AWDLoadTrqnsGain_c]  "VTQD_AWDLoadTrqnsGain_c"
  [VTQD_AWDLoadTrqnsGain_c] -> Product/2
  VTQD_EstVehWeightResult_kg/1 -> [VTQD_EstVehWeightResult_kg]
  [VTQD_EstVehWeightResult_kg] -> MTQD_AWDLoadTrqnsGain_Z_c/2
  LiuzgSwitch2/1 -> LiuzgSwitch4/3
  [VINP_DriverSelPowerTrain_enum] -> Equal1/1
  Constant4/1 -> Equal1/2
  LiuzgSwitch5/1 -> LiuzgSwitch4/1
  Constant3/1 -> Equal3/2
  [VINP_DriverSelPowerTrain_enum] -> Equal3/1
  Equal3/1 -> LiuzgSwitch5/2
  LiuzgSwitch4/1 -> Saturation/1
  Constant7/1 -> LiuzgSwitch5/3
  Constant6/1 -> LiuzgSwitch5/1
  Ground/1 -> [VINP_DriverSelPowerTrain_enum]  "VINP_DriverSelPowerTrain_enum"
  Subtract/1 -> Switch/3
  Switch/1 -> VTQD_FrRatio_AWD/1  "VTQD_FrEDUSpRat_rat"
  Switch1/1 -> VTQD_RrRatio_AWD/1  "VTQD_RrEDUSpRat_rat"
  Constant8/1 -> Switch/2
  Constant9/1 -> Switch/1
  Constant11/1 -> Switch1/1
  Constant10/1 -> Switch1/2
  Constant12/1 -> AND/2
  Equal1/1 -> AND/1
  AND/1 -> LiuzgSwitch4/2
  VVMC_ActRRSlideRate_pct/1 -> [VVMC_ActRRSlideRate_pct]
  VVMC_ActLRSlideRate_pct/1 -> [VVMC_ActLRSlideRate_pct]
  [VVMC_ActLRSlideRate_pct] -> Abs/1
  [VVMC_ActRRSlideRate_pct] -> Abs1/1
  Abs1/1 -> Max/2
  Abs/1 -> Max/1
  Max/1 -> MTQD_AWDLoadTrqnsGain_Z_c/1  "VTQD_AWDLoadTrqnsGain_pct"
  Constant13/1 -> Switch2/2
  VVMC_RearTqRatio_rat/1 -> Switch2/1
  Switch2/1 -> LiuzgSwitch2/3
  OR1/1 -> LiuzgSwitch2/2
  Constant14/1 -> NOT/1
  NOT/1 -> OR1/2

== system tqd/TQD/TorqueDemand/TorqueModule/TqDistribution/FWD_Ratio ==
  Action Port : ActionPort
  Constant : Constant  Value=ONE_FLOAT
  Constant1 : Constant  Value=ZERO_FLOAT
  VTQD_FrRatio_FWD : Outport
  VTQD_RrRatio_FWD : Outport  Port=2
  wires:
  Constant/1 -> VTQD_FrRatio_FWD/1
  Constant1/1 -> VTQD_RrRatio_FWD/1

== system tqd/TQD/TorqueDemand/TorqueModule/TqDistribution/RWD_Ratio ==
  Action Port : ActionPort
  Constant : Constant  Value=ONE_FLOAT
  Constant1 : Constant  Value=ZERO_FLOAT
  VTQD_FrRatio_RWD : Outport
  VTQD_RrRatio_RWD : Outport  Port=2
  wires:
  Constant1/1 -> VTQD_FrRatio_RWD/1
  Constant/1 -> VTQD_RrRatio_RWD/1

== system tqd/TQD/TorqueDemand/Signal_convert/VehWeightEst/Calaulation/Front Wheel Torque ==
  VINP_FrEDURealTMTq_Nm : Inport
  VTQD_VehWeightEstEn_flg : Inport  Port=2
  VTQD_VehWeightEstDis_flg : Inport  Port=3
  VTQD_VehWeightEstEnd_flg : Inport  Port=4
  task_time_s : Inport  Port=5
  AND : Logic  AllPortsSameDT=off  OutDataTypeStr=boolean
  AND1 : Logic  AllPortsSameDT=off  OutDataTypeStr=boolean
  AND2 : Logic  AllPortsSameDT=off  OutDataTypeStr=boolean
  Abs : Abs
  Add : Sum
  Add1 : Sum
  Add2 : Sum  Inputs=+-
  Constant1 : Constant  Value=ZERO_FLOAT
  Constant2 : Constant  Value=KTQD_VehWeighEstTime_s
  Constant3 : Constant  Value=ZERO_FLOAT
  Constant4 : Constant  Value=KTQD_VehWeighEstTimeTune_cnt
  Constant5 : Constant  Value=ZERO_FLOAT
  Constant6 : Constant  Value=KTQD_EstFrWhlTqDev_Nm
  Data Type Conversion : DataTypeConversion  OutDataTypeStr=uint8
  Delay{,1..4} (5 alike) : Delay  DelayLength=1
  Detect Decrease : simulink/Logic and Bit Operations/Detect Decrease  vinit=0.0  OutDataTypeStr=boolean
  Detect Increase : simulink/Logic and Bit Operations/Detect Increase  vinit=0.0  OutDataTypeStr=boolean
  Divide : Product  Inputs=*/
  Divide1 : Product  Inputs=*/
  Min : MinMax  Inputs=2
  NOT : Logic  Operator=NOT  AllPortsSameDT=off  OutDataTypeStr=boolean
  NOT1 : Logic  Operator=NOT  AllPortsSameDT=off  OutDataTypeStr=boolean
  Relational Operator : RelationalOperator  Operator=<=  OutDataTypeStr=boolean  RndMeth=Simplest
  Switch{,1..3} (4 alike) : Switch  Criteria=u2 > Threshold
  Terminator : Terminator
  VTQD_EstFrRealTqAvg_Nm : Outport
  VTQD_EstFrRealTqCheckPass_flg : Outport  Port=2
  wires:
  task_time_s/1 -> [task_time_s]
  VTQD_VehWeightEstEnd_flg/1 -> Terminator/1
  VTQD_VehWeightEstDis_flg/1 -> [VTQD_VehWeightEstDis_flg]
  VTQD_VehWeightEstEn_flg/1 -> [VTQD_VehWeightEstEn_flg]
  VINP_FrEDURealTMTq_Nm/1 -> [VINP_FrEDURealTMTq_Nm]
  AND1/1 -> [VTQD_EstFrRealTqCheckPass_flg]  "VTQD_EstFrRealTqCheckPass_flg"
  [VTQD_VehWeightEstDis_flg] -> AND1/1
  Add2/1 -> Abs/1
  Abs/1 -> Relational Operator/1
  Delay/1 -> NOT/1
  Detect Increase/1 -> Switch2/2
  [task_time_s] -> Divide/2
  [VTQD_EstFrRealTqMin_Nm] -> Delay2/1
  Delay2/1 -> Min/2
  [VTQD_VehWeightEstDis_flg] -> Delay/1
  [VTQD_EstFrRealTqMin_Nm] -> Add2/2
  Constant2/1 -> Divide/1
  Switch2/1 -> Delay4/1, [VTQD_EstFrRealTqMin_Nm]  "VTQD_EstFrRealTqMin_Nm"
  Add1/1 -> Divide1/2  "VTQD_EstCycleCount_cnt"
  Switch1/1 -> Delay1/1, [VTQD_EstFrRealTqSum_Nm]  "VTQD_EstFrRealTqSum_Nm"
  Constant5/1 -> Switch1/1
  NOT/1 -> AND/2
  [VINP_FrEDURealTMTq_Nm] -> Switch/1
  [VTQD_EstFrRealTqAvg_Nm] -> Add2/1
  Constant6/1 -> Relational Operator/2
  Add/1 -> Switch1/3
  Relational Operator/1 -> AND1/2
  [VTQD_VehWeightEstEn_flg] -> Detect Increase/1
  Constant1/1 -> Switch/3
  AND/1 -> Switch/2
  [VTQD_VehWeightEstEn_flg] -> Detect Decrease/1
  [VTQD_EstFrRealTqSum_Nm] -> Divide1/1
  Divide/1 -> Data Type Conversion/1
  Switch/1 -> Add/1
  Divide1/1 -> [VTQD_EstFrRealTqAvg_Nm]  "VTQD_EstFrRealTqAvg_Nm"
  [VTQD_VehWeightEstEn_flg] -> AND/1
  Constant3/1 -> Switch2/1
  Delay1/1 -> Add/2
  [VINP_FrEDURealTMTq_Nm] -> Min/1
  Constant4/1 -> Add1/2
  [VTQD_EstFrRealTqCheckPass_flg] -> VTQD_EstFrRealTqCheckPass_flg/1
  [VTQD_EstFrRealTqAvg_Nm] -> VTQD_EstFrRealTqAvg_Nm/1
  Data Type Conversion/1 -> Add1/1
  Delay3/1 -> NOT1/1
  [VTQD_VehWeightEstEn_flg] -> AND2/1
  AND2/1 -> Switch3/2
  NOT1/1 -> AND2/2
  [VTQD_VehWeightEstDis_flg] -> Delay3/1
  Delay4/1 -> Switch3/3
  Min/1 -> Switch3/1
  Switch3/1 -> Switch2/3
  Detect Decrease/1 -> Switch1/2

== system tqd/TQD/TorqueDemand/Signal_convert/VehWeightEst/Calaulation/Long Acc ==
  VVMC_LongAcc_Gps : Inport
  VTQD_VehWeightEstEn_flg : Inport  Port=2
  VTQD_VehWeightEstDis_flg : Inport  Port=3
  VTQD_VehWeightEstEnd_flg : Inport  Port=4
  task_time_s : Inport  Port=5
  AND : Logic  AllPortsSameDT=off  OutDataTypeStr=boolean
  AND1 : Logic  AllPortsSameDT=off  OutDataTypeStr=boolean
  AND2 : Logic  AllPortsSameDT=off  OutDataTypeStr=boolean
  Abs : Abs
  Abs1 : Abs
  Add : Sum
  Add1 : Sum
  Add2 : Sum  Inputs=+-
  Constant1 : Constant  Value=ZERO_FLOAT
  Constant2 : Constant  Value=KTQD_VehWeighEstTime_s
  Constant3 : Constant  Value=ZERO_FLOAT
  Constant4 : Constant  Value=KTQD_VehWeighEstTimeTune_cnt
  Constant5 : Constant  Value=ZERO_FLOAT
  Constant6 : Constant  Value=KTQD_EstLongAccDev_Gps
  Constant7 : Constant  Value=KTQD_VehWeighEstIntAcc_Gps
  Constant8 : Constant  Value=KTQD_VehWeighEstIntAcc_Gps
  Data Type Conversion : DataTypeConversion  OutDataTypeStr=uint8
  Delay{,1..4} (5 alike) : Delay  DelayLength=1
  Detect Decrease : simulink/Logic and Bit Operations/Detect Decrease  vinit=0.0  OutDataTypeStr=boolean
  Detect Increase : simulink/Logic and Bit Operations/Detect Increase  vinit=0.0  OutDataTypeStr=boolean
  Divide : Product  Inputs=*/
  Divide1 : Product  Inputs=*/
  Min : MinMax  Inputs=2
  NOT : Logic  Operator=NOT  AllPortsSameDT=off  OutDataTypeStr=boolean
  NOT1 : Logic  Operator=NOT  AllPortsSameDT=off  OutDataTypeStr=boolean
  Relational Operator : RelationalOperator  Operator=<=  OutDataTypeStr=boolean  RndMeth=Simplest
  Relational Operator1 : RelationalOperator  Operator=<=  OutDataTypeStr=boolean  RndMeth=Simplest
  Switch{,1..4} (5 alike) : Switch  Criteria=u2 > Threshold
  Terminator : Terminator
  VTQD_EstLongAccAvg_Gps : Outport
  VTQD_EstLongAccCheckPass_flg : Outport  Port=2
  wires:
  Constant4/1 -> Add1/2
  [VVMC_LongAcc_Gps] -> Min/1
  Delay1/1 -> Add/2
  Constant3/1 -> Switch2/1
  [VTQD_VehWeightEstEn_flg] -> AND/1
  Divide1/1 -> [VTQD_EstLongAccAvg_Gps]  "VTQD_EstLongAccAvg_Gps"
  Switch/1 -> Add/1
  Data Type Conversion/1 -> Add1/1
  AND/1 -> Switch/2
  Constant1/1 -> Switch/3
  [VTQD_VehWeightEstEn_flg] -> Detect Increase/1
  Relational Operator/1 -> AND1/2
  Divide/1 -> Data Type Conversion/1
  Add/1 -> Switch1/3
  Constant6/1 -> Relational Operator/2
  [VTQD_EstLongAccAvg_Gps] -> Add2/1
  [VVMC_LongAcc_Gps] -> Switch/1
  NOT/1 -> AND/2
  Constant5/1 -> Switch1/1
  Switch1/1 -> [VTQD_EstLongAccSum_Gps], Delay1/1  "VTQD_EstLongAccSum_Gps"
  Add1/1 -> Divide1/2  "VTQD_EstCycleCount_cnt"
  Switch2/1 -> Delay4/1, [VTQD_EstLongAccMin_Gps]  "VTQD_EstLongAccMin_Gps"
  Constant2/1 -> Divide/1
  [VTQD_EstLongAccMin_Gps] -> Add2/2
  [VTQD_VehWeightEstDis_flg] -> Delay/1
  Delay2/1 -> Min/2
  [VTQD_EstLongAccMin_Gps] -> Delay2/1
  [task_time_s] -> Divide/2
  Detect Increase/1 -> Switch2/2
  Delay/1 -> NOT/1
  Abs/1 -> Relational Operator/1
  Add2/1 -> Abs/1
  [VTQD_VehWeightEstDis_flg] -> AND1/1
  AND1/1 -> [VTQD_EstLongAccCheckPass_flg]  "VTQD_EstLongAccCheckPass_flg"
  VVMC_LongAcc_Gps/1 -> [VVMC_LongAcc_Gps]
  VTQD_VehWeightEstEn_flg/1 -> [VTQD_VehWeightEstEn_flg]
  VTQD_VehWeightEstDis_flg/1 -> [VTQD_VehWeightEstDis_flg]
  VTQD_VehWeightEstEnd_flg/1 -> Terminator/1
  task_time_s/1 -> [task_time_s]
  [VTQD_EstLongAccAvg_Gps] -> VTQD_EstLongAccAvg_Gps/1
  [VTQD_EstLongAccCheckPass_flg] -> VTQD_EstLongAccCheckPass_flg/1
  AND2/1 -> Switch3/2
  [VTQD_VehWeightEstDis_flg] -> Delay3/1
  NOT1/1 -> AND2/2
  [VTQD_VehWeightEstEn_flg] -> AND2/1
  Delay3/1 -> NOT1/1
  Min/1 -> Switch3/1
  Delay4/1 -> Switch3/3
  Switch3/1 -> Switch2/3
  Detect Decrease/1 -> Switch1/2
  [VTQD_VehWeightEstEn_flg] -> Detect Decrease/1
  [VTQD_EstLongAccSum_Gps] -> Switch4/3
  Switch4/1 -> Divide1/1
  [VTQD_EstLongAccSum_Gps] -> Abs1/1
  Abs1/1 -> Relational Operator1/1
  Relational Operator1/1 -> Switch4/2
  Constant7/1 -> Relational Operator1/2
  Constant8/1 -> Switch4/1

== system tqd/TQD/TorqueDemand/Signal_convert/VehWeightEst/Calaulation/Rear Wheel Torque ==
  VINP_RrEDURealTMTq_Nm : Inport
  VTQD_VehWeightEstEn_flg : Inport  Port=2
  VTQD_VehWeightEstDis_flg : Inport  Port=3
  VTQD_VehWeightEstEnd_flg : Inport  Port=4
  task_time_s : Inport  Port=5
  AND : Logic  AllPortsSameDT=off  OutDataTypeStr=boolean
  AND1 : Logic  AllPortsSameDT=off  OutDataTypeStr=boolean
  AND2 : Logic  AllPortsSameDT=off  OutDataTypeStr=boolean
  Abs : Abs
  Add : Sum
  Add1 : Sum
  Add2 : Sum  Inputs=+-
  Constant1 : Constant  Value=ZERO_FLOAT
  Constant2 : Constant  Value=KTQD_VehWeighEstTime_s
  Constant3 : Constant  Value=ZERO_FLOAT
  Constant4 : Constant  Value=KTQD_VehWeighEstTimeTune_cnt
  Constant5 : Constant  Value=ZERO_FLOAT
  Constant6 : Constant  Value=KTQD_EstRrWhlTqDev_Nm
  Data Type Conversion : DataTypeConversion  OutDataTypeStr=uint8
  Delay{,1..4} (5 alike) : Delay  DelayLength=1
  Detect Decrease : simulink/Logic and Bit Operations/Detect Decrease  vinit=0.0  OutDataTypeStr=boolean
  Detect Increase : simulink/Logic and Bit Operations/Detect Increase  vinit=0.0  OutDataTypeStr=boolean
  Divide : Product  Inputs=*/
  Divide1 : Product  Inputs=*/
  Min : MinMax  Inputs=2
  NOT : Logic  Operator=NOT  AllPortsSameDT=off  OutDataTypeStr=boolean
  NOT1 : Logic  Operator=NOT  AllPortsSameDT=off  OutDataTypeStr=boolean
  Relational Operator : RelationalOperator  Operator=<=  OutDataTypeStr=boolean  RndMeth=Simplest
  Switch{,1..3} (4 alike) : Switch  Criteria=u2 > Threshold
  Terminator : Terminator
  VTQD_EstRrRealTqAvg_Nm : Outport
  VTQD_EstRrRealTqCheckPass_flg : Outport  Port=2
  wires:
  [VTQD_EstRrRealTqAvg_Nm] -> VTQD_EstRrRealTqAvg_Nm/1
  [VTQD_EstRrRealTqCheckPass_flg] -> VTQD_EstRrRealTqCheckPass_flg/1
  Constant4/1 -> Add1/2
  [VINP_RrEDURealTMTq_Nm] -> Min/1
  Delay1/1 -> Add/2
  Constant3/1 -> Switch2/1
  [VTQD_VehWeightEstEn_flg] -> AND/1
  Divide1/1 -> [VTQD_EstRrRealTqAvg_Nm]  "VTQD_EstRrRealTqAvg_Nm"
  Switch/1 -> Add/1
  [VTQD_EstRrRealTqSum_Nm] -> Divide1/1
  [VTQD_VehWeightEstEn_flg] -> Detect Decrease/1
  AND/1 -> Switch/2
  Constant1/1 -> Switch/3
  [VTQD_VehWeightEstEn_flg] -> Detect Increase/1
  Relational Operator/1 -> AND1/2
  Add/1 -> Switch1/3
  Constant6/1 -> Relational Operator/2
  [VTQD_EstRrRealTqAvg_Nm] -> Add2/1
  [VINP_RrEDURealTMTq_Nm] -> Switch/1
  NOT/1 -> AND/2
  Constant5/1 -> Switch1/1
  Switch1/1 -> [VTQD_EstRrRealTqSum_Nm], Delay1/1  "VTQD_EstRrRealTqSum_Nm"
  Switch2/1 -> Delay4/1, [VTQD_EstRrRealTqMin_Nm]  "VTQD_EstRrRealTqMin_Nm"
  Constant2/1 -> Divide/1
  [VTQD_EstRrRealTqMin_Nm] -> Add2/2
  [VTQD_VehWeightEstDis_flg] -> Delay/1
  Delay2/1 -> Min/2
  [VTQD_EstRrRealTqMin_Nm] -> Delay2/1
  [task_time_s] -> Divide/2
  Detect Increase/1 -> Switch2/2
  Delay/1 -> NOT/1
  Abs/1 -> Relational Operator/1
  Add2/1 -> Abs/1
  [VTQD_VehWeightEstDis_flg] -> AND1/1
  AND1/1 -> [VTQD_EstRrRealTqCheckPass_flg]  "VTQD_EstRrRealTqCheckPass_flg"
  VINP_RrEDURealTMTq_Nm/1 -> [VINP_RrEDURealTMTq_Nm]
  VTQD_VehWeightEstEn_flg/1 -> [VTQD_VehWeightEstEn_flg]
  VTQD_VehWeightEstDis_flg/1 -> [VTQD_VehWeightEstDis_flg]
  VTQD_VehWeightEstEnd_flg/1 -> Terminator/1
  task_time_s/1 -> [task_time_s]
  Add1/1 -> Divide1/2  "VTQD_EstCycleCount_cnt"
  Divide/1 -> Data Type Conversion/1
  Data Type Conversion/1 -> Add1/1
  [VTQD_VehWeightEstEn_flg] -> AND2/1
  NOT1/1 -> AND2/2
  Delay3/1 -> NOT1/1
  [VTQD_VehWeightEstDis_flg] -> Delay3/1
  AND2/1 -> Switch3/2
  Min/1 -> Switch3/1
  Switch3/1 -> Switch2/3
  Delay4/1 -> Switch3/3
  Detect Decrease/1 -> Switch1/2

== system tqd/TQD/TorqueDemand/Signal_convert/VehWeightEst/Calaulation/Vehicle Weight ==
  VTQD_EstFrRealTqAvg_Nm : Inport
  VTQD_EstRrRealTqAvg_Nm : Inport  Port=2
  VTQD_EstLongAccAvg_Gps : Inport  Port=3
  VINP_VehSpeed_kph : Inport  Port=4
  Add : Sum  Inputs=+++
  Add1 : Sum
  Add2 : Sum
  Add3 : Sum
  Constant1 : Constant  Value=KTQD_RrTMTotalGearRatio_gain
  Constant10 : Constant  Value=KTQR_FrTMGearEff_c
  Constant11 : Constant  Value=KTQR_RrTMGearEff_c
  Constant12 : Constant  Value=MINUSONE_FLOAT
  Constant13 : Constant  Value=KTQD_GravityValue_mps2
  Constant2 : Constant  Value=KTQD_FrTMTotalGearRatio_gain
  Constant3 : Constant  Value=MINUSONE_FLOAT
  Constant4 : Constant  Value=MINUSONE_FLOAT
  Constant5 : Constant  Value=KTQD_FrTireRadius_m
  Constant6 : Constant  Value=KTQD_RrTireRadius_m
  Constant7 : Constant  Value=KTQD_EstRollCoeffA_c
  Constant8 : Constant  Value=KTQD_EstRollCoeffB_c
  Constant9 : Constant  Value=KTQD_EstRollCoeffC_c
  Divide : Product  Inputs=*/
  Divide1 : Product  Inputs=*/
  Divide2 : Product  Inputs=*/
  Product{,3..5} (4 alike) : Product
  Product1 : Product  Inputs=3
  Product2 : Product  Inputs=3
  Product6 : Product  Inputs=3
  Square : Math  Operator=square  SaturateOnIntegerOverflow=on
  VTQD_EstVehWeight_kg : Outport
  wires:
  [VINP_VehSpeed_kph] -> Square/1
  Divide/1 -> Add1/1  "VTQD_EstFrForce_N"
  Product2/1 -> Divide2/1  "VTQD_EstRrWhlTqAvg_Nm"
  [VINP_VehSpeed_kph] -> Product/2
  Constant6/1 -> Divide2/2
  Product1/1 -> Divide/1  "VTQD_EstFrWhlTqAvg_Nm"
  Constant2/1 -> Product1/2
  Constant1/1 -> Product2/2
  Add1/1 -> Product4/1
  Square/1 -> Product3/2
  [VTQD_EstRrRealTqAvg_Nm] -> Product2/1
  Constant3/1 -> Product1/3
  [VTQD_EstRollForce_N] -> Add2/2
  Constant9/1 -> Product3/1
  Constant7/1 -> Add/1
  [VTQD_EstFrRealTqAvg_Nm] -> Product1/1
  Constant10/1 -> Product4/2
  Add2/1 -> Product5/1
  Product4/1 -> Add3/1  "VTQD_EstFrActForce_N"
  Constant5/1 -> Divide/2
  Add/1 -> [VTQD_EstRollForce_N]  "VTQD_EstRollForce_N"
  Product/1 -> Add/2
  Constant4/1 -> Product2/3
  Add3/1 -> [VTQD_EstActTotalForce_N]  "VTQD_EstActTotalForce_N"
  Product5/1 -> Add3/2  "VTQD_EstRrActForce_N"
  Constant8/1 -> Product/1
  Divide2/1 -> Add2/1  "VTQD_EstRrForce_N"
  Constant11/1 -> Product5/2
  [VTQD_EstRollForce_N] -> Add1/2
  Product3/1 -> Add/3
  [VTQD_EstLongAccAvg_Gps] -> Product6/1
  Constant12/1 -> Product6/2
  Product6/1 -> Divide1/2
  [VTQD_EstActTotalForce_N] -> Divide1/1
  VTQD_EstFrRealTqAvg_Nm/1 -> [VTQD_EstFrRealTqAvg_Nm]
  VTQD_EstRrRealTqAvg_Nm/1 -> [VTQD_EstRrRealTqAvg_Nm]
  VTQD_EstLongAccAvg_Gps/1 -> [VTQD_EstLongAccAvg_Gps]
  VINP_VehSpeed_kph/1 -> [VINP_VehSpeed_kph]
  [VTQD_EstVehWeight_kg] -> VTQD_EstVehWeight_kg/1
  Constant13/1 -> Product6/3
  Divide1/1 -> [VTQD_EstVehWeight_kg]  "VTQD_EstVehWeight_kg"

== system tqd/TQD/TorqueDemand/TorqueModule/AvaliableTqLimit/TorqueCapacityCalcalation/CapacityDistribution ==
  VTQD_FrEDUSpRat_cmd : Inport
  VTQD_RrEDUSpRat_rat : Inport  Port=2
  VTQD_TMPwrAvailDchrg_kW : Inport  Port=3
  VINP_HVBPwrAvailChrg_kw : Inport  Port=4
  Abs1 : Abs
  Product{,1,4..5} (4 alike) : Product
  VTQD_FrHVBPwrAvailDchrg_kw : Outport
  VTQD_RrHVBPwrAvailDchrg_kw : Outport  Port=2
  VTQD_FrHVBPwrAvailChrg_kw : Outport  Port=3
  VTQD_RrHVBPwrAvailChrg_kw : Outport  Port=4
  wires:
  VTQD_RrEDUSpRat_rat/1 -> [VTQD_RrEDUSpRat_rat]
  VTQD_FrEDUSpRat_cmd/1 -> [VTQD_FrEDUSpRat_rat]
  VINP_HVBPwrAvailChrg_kw/1 -> Abs1/1
  Product4/1 -> VTQD_FrHVBPwrAvailChrg_kw/1
  Product5/1 -> VTQD_RrHVBPwrAvailChrg_kw/1
  Product1/1 -> VTQD_RrHVBPwrAvailDchrg_kw/1  "VTQD_RrHVBPwrAvailDchrg_kW"
  [VTQD_FrEDUSpRat_rat] -> Product4/1
  [VTQD_FrEDUSpRat_rat] -> Product/1
  Abs1/1 -> Product4/2, Product5/1
  VTQD_TMPwrAvailDchrg_kW/1 -> Product1/1, Product/2
  [VTQD_RrEDUSpRat_rat] -> Product5/2
  Product/1 -> VTQD_FrHVBPwrAvailDchrg_kw/1  "VTQD_FrHVBPwrAvailDchrg_kW"
  [VTQD_RrEDUSpRat_rat] -> Product1/2

== system tqd/TQD/TorqueDemand/TorqueModule/AvaliableTqLimit/TorqueCapacityCalcalation/Generation ==
  VTQD_FrShaftSpd_rpm : Inport
  VTQD_RrShaftSpd_rpm : Inport  Port=2
  VTQD_FrHVBPwrAvailChrg_kw : Inport  Port=3
  VTQD_RrHVBPwrAvailChrg_kw : Inport  Port=4
  KTQD_FrBatapCont_factor : Inport  Port=5
  KTQD_RrBatapCont_factor : Inport  Port=6
  Abs2 : Abs
  Abs6 : Abs
  Constant : Constant  Value=KTQD_WhlTqCap_ovrdflg
  Constant1 : Constant  Value=KTQD_WhlTqCapGen_ovrdval
  Constant2 : Constant  Value=KTQD_RrTMSpdMin_rpm  OutDataTypeStr=single
  Constant3 : Constant  Value=KTQD_WhlTqCap_ovrdflg
  Constant5 : Constant  Value=KTQD_FrTMSpdMin_rpm  OutDataTypeStr=single
  Constant7 : Constant  Value=KTQD_WhlTqCapGen_ovrdval
  Fcn : Fcn  Expr=u[1]/u[2]/pi*u[3]
  Fcn2 : Fcn  Expr=u[1]/u[2]/pi*u[3]
  Gain1 : Gain  Gain=-1
  Gain4 : Gain  Gain=-1
  Max1 : MinMax  Function=max  Inputs=2
  Max4 : MinMax  Function=max  Inputs=2
  Mux : Mux  Inputs=3
  Mux2 : Mux  Inputs=3
  Saturation1 : Saturate  UpperLimit=0  LowerLimit=KTQD_FrLowTheldTrq_Nm
      settings: AttributesFormatString=|
      | Upper Limit :%<UpperLimit>
      | Lower Limit :%<LowerLimit>
  Saturation2 : Saturate  UpperLimit=0  LowerLimit=KTQD_RrLowTheldTrq_Nm
      settings: AttributesFormatString=|
      | Upper Limit :%<UpperLimit>
      | Lower Limit :%<LowerLimit>
  Switch : Switch  Criteria=u2 ~= 0
      settings: AttributesFormatString=<%<Criteria>>
  Switch1 : Switch  Criteria=u2 ~= 0
      settings: AttributesFormatString=<%<Criteria>>
  VTQD_WhlTqCapGenFr_Nm : Outport
  VTQD_WhlTqCapGenRr_Nm : Outport  Port=2
  wires:
  Gain1/1 -> Saturation2/1
  Gain4/1 -> Saturation1/1
  Saturation2/1 -> Switch1/3
  Switch1/1 -> VTQD_WhlTqCapGenRr_Nm/1  "VTQD_WhlTqCapGenRr_Nm"
  Constant3/1 -> Switch1/2
  Constant7/1 -> Switch1/1
  Saturation1/1 -> Switch/3
  Switch/1 -> VTQD_WhlTqCapGenFr_Nm/1  "VTQD_WhlTqCapGenFr_Nm"
  Constant1/1 -> Switch/1
  Constant/1 -> Switch/2
  VTQD_RrHVBPwrAvailChrg_kw/1 -> [VTQD_RrHVBPwrAvailChrg_kw]
  KTQD_FrBatapCont_factor/1 -> [KTQD_FrBatapCont_factor]
  VTQD_FrHVBPwrAvailChrg_kw/1 -> [VTQD_FrHVBPwrAvailChrg_kw]
  VTQD_FrShaftSpd_rpm/1 -> [VTQD_FrShaftSpd_rpm]
  VTQD_RrShaftSpd_rpm/1 -> [VTQD_RrShaftSpd_rpm]
  KTQD_RrBatapCont_factor/1 -> [KTQD_RrBatapCont_factor]
  Fcn2/1 -> Gain1/1
  Max1/1 -> Mux2/2
  Abs2/1 -> Max1/1
  Mux2/1 -> Fcn2/1
  Constant2/1 -> Max1/2
  [KTQD_RrBatapCont_factor] -> Mux2/3
  [VTQD_RrShaftSpd_rpm] -> Abs2/1
  [VTQD_RrHVBPwrAvailChrg_kw] -> Mux2/1
  Fcn/1 -> Gain4/1
  Abs6/1 -> Max4/1
  [VTQD_FrHVBPwrAvailChrg_kw] -> Mux/1
  Constant5/1 -> Max4/2
  [VTQD_FrShaftSpd_rpm] -> Abs6/1
  [KTQD_FrBatapCont_factor] -> Mux/3
  Mux/1 -> Fcn/1
  Max4/1 -> Mux/2

== system tqd/TQD/TorqueDemand/TorqueModule/AvaliableTqLimit/TorqueCapacityCalcalation/Motoring ==
  VTQD_FrShaftSpd_rpm : Inport
  VTQD_RrShaftSpd_rpm : Inport  Port=2
  VTQD_FrHVBPwrAvailDchrg_kw : Inport  Port=3
  VTQD_RrHVBPwrAvailDchrg_kw : Inport  Port=4
  KTQD_FrBatapCont_factor : Inport  Port=5
  KTQD_RrBatapCont_factor : Inport  Port=6
  VINP_HVBCellVoltMax_mV : Inport  Port=7
  VINP_HVBCellVoltMin_mV : Inport  Port=8
  VINP_HVBSOH_pct : Inport  Port=9
  Abs : Abs
  Abs2 : Abs
  Add : Sum  Commented=on  Inputs=+-
  Constant : Constant  Value=KTQD_WhlTqCap_ovrdflg
  Constant1 : Constant  Value=KTQD_FrTMSpdMin_rpm  OutDataTypeStr=single
  Constant2 : Constant  Value=ZERO_FLOAT
  Constant3 : Constant  Value=KTQD_RrTMSpdMin_rpm  OutDataTypeStr=single
  Constant4 : Constant  Value=ZERO_FLOAT
  Constant5 : Constant  Value=KTQD_WhlTqCapMot_ovrdval
  Constant6 : Constant  Value=KTQD_WhlTqCap_ovrdflg
  Constant7 : Constant  Value=KTQD_WhlTqCapMot_ovrdval
  Constant8 : Constant  Value=KTQD_FrUppTheldTrq_Nm
  Constant9 : Constant  Value=KTQD_RrUppTheldTrq_Nm
  Fcn : Fcn  Expr=u[1]/u[2]/pi*u[3]
  Fcn2 : Fcn  Expr=u[1]/u[2]/pi*u[3]
  From3 : From  Commented=on  GotoTag=VINP_HVBCellVoltMax_mV
  From4 : From  Commented=on  GotoTag=VINP_HVBCellVoltMin_mV
  From5 : From  Commented=on  GotoTag=VTQD_HCBCellVoltDev_mV
  From6 : From  Commented=on  GotoTag=VINP_HVBSOH_pct
  Goto7 : Goto  Commented=on  GotoTag=VTQD_HCBCellVoltDev_mV
  Goto9 : Goto  Commented=on  GotoTag=VTQD_WhlTqCapMotGain_c
  MTQD_WhlTqCapMotGain_Z_c : Lookup_n-D  Commented=on  BreakpointsForDimension1=ATQD_WhlTqCapMotGain_Y_mV  BreakpointsForDimension2=ATQD_WhlTqCapMotGain_X_pct  Table=MTQD_WhlTqCapMotGain_Z_c  InternalRulePriority=Speed  RndMeth=Simplest  InputSameDT=on
      settings: InputPortMap=u0,u1
  Max{,1..3} (4 alike) : MinMax  Function=max  Inputs=2
  Min : MinMax  Inputs=2
  Min1 : MinMax  Inputs=2
  Mux : Mux  Inputs=3
  Mux2 : Mux  Inputs=3
  Switch : Switch  Criteria=u2 ~= 0
      settings: AttributesFormatString=<%<Criteria>>
  Switch1 : Switch  Criteria=u2 ~= 0
      settings: AttributesFormatString=<%<Criteria>>
  VTQD_WhlTqCapMotFr_Nm : Outport
  VTQD_WhlTqCapMotRr_Nm : Outport  Port=2
  wires:
  Fcn2/1 -> Min1/1
  Switch1/1 -> VTQD_WhlTqCapMotRr_Nm/1  "VTQD_WhlTqCapMotRr_Nm"
  Constant7/1 -> Switch1/1
  Constant6/1 -> Switch1/2
  Constant5/1 -> Switch/1
  Constant/1 -> Switch/2
  Switch/1 -> VTQD_WhlTqCapMotFr_Nm/1  "VTQD_WhlTqCapMotFr_Nm"
  VTQD_RrHVBPwrAvailDchrg_kw/1 -> [VTQD_RrHVBPwrAvailDchrg_kw]
  KTQD_RrBatapCont_factor/1 -> [KTQD_RrBatapCont_factor]
  VTQD_RrShaftSpd_rpm/1 -> [VTQD_RrShaftSpd_rpm]
  Abs2/1 -> Max2/1
  [VTQD_RrHVBPwrAvailDchrg_kw] -> Mux2/1
  Constant3/1 -> Max2/2
  [VTQD_RrShaftSpd_rpm] -> Abs2/1
  Mux2/1 -> Fcn2/1
  Max2/1 -> Mux2/2
  [VTQD_FrHVBPwrAvailDchrg_kw] -> Mux/1
  Max/1 -> Mux/2
  [VTQD_FrShaftSpd_rpm] -> Abs/1
  KTQD_FrBatapCont_factor/1 -> [KTQD_FrBatapCont_factor]
  VTQD_FrHVBPwrAvailDchrg_kw/1 -> [VTQD_FrHVBPwrAvailDchrg_kw]
  Abs/1 -> Max/1
  Fcn/1 -> Min/1
  Mux/1 -> Fcn/1
  VTQD_FrShaftSpd_rpm/1 -> [VTQD_FrShaftSpd_rpm]
  Constant1/1 -> Max/2
  Constant8/1 -> Min/2
  Min/1 -> Max1/1
  Constant2/1 -> Max1/2
  Constant9/1 -> Min1/2
  Min1/1 -> Max3/1
  Constant4/1 -> Max3/2
  VINP_HVBCellVoltMin_mV/1 -> [VINP_HVBCellVoltMin_mV]
  VINP_HVBSOH_pct/1 -> [VINP_HVBSOH_pct]
  VINP_HVBCellVoltMax_mV/1 -> [VINP_HVBCellVoltMax_mV]
  Add/1 -> Goto7/1  "VTQD_HCBCellVoltDev_mV"
  From3/1 -> Add/1
  From4/1 -> Add/2
  From5/1 -> MTQD_WhlTqCapMotGain_Z_c/1
  [KTQD_FrBatapCont_factor] -> Mux/3
  [KTQD_RrBatapCont_factor] -> Mux2/3
  MTQD_WhlTqCapMotGain_Z_c/1 -> Goto9/1  "VTQD_WhlTqCapMotGain_c"
  Max1/1 -> Switch/3
  Max3/1 -> Switch1/3
  From6/1 -> MTQD_WhlTqCapMotGain_Z_c/2

== system tqd/TQD/TorqueDemand/TorqueModule/AvaliableTqLimit/TorqueCapacityCalcalation/TMAvailablePwr_Calculation ==
  VINP_HVBPwrAvailDchrg_kw : Inport
  Add : Sum
  Constant : Constant  Value=KTQD_DCDCCalPwrAvailRsv_kW
  Constant1 : Constant  Value=KTQD_THCMCalPwrAvailRsv_kW
  Constant2 : Constant  Value=KTQD_TMPwrAvailDchrg_kW_ovrdflg
  Constant3 : Constant  Value=ZERO_FLOAT
  Min : MinMax  Function=max  Inputs=2
  Subtract : Sum  Inputs=+-
  Switch : Switch  Criteria=u2 ~= 0
      settings: AttributesFormatString=<%<Criteria>>
  VTQD_TMPwrAvailDchrg_kW : Outport
  wires:
  Constant3/1 -> Min/2
  Min/1 -> Switch/1
  Switch/1 -> VTQD_TMPwrAvailDchrg_kW/1  "VTQD_TMPwrAvailDchrg_kW"
  Constant2/1 -> Switch/2
  Subtract/1 -> Min/1
  Add/1 -> Subtract/2
  VINP_HVBPwrAvailDchrg_kw/1 -> Subtract/1, Switch/3
  Constant1/1 -> Add/2
  Constant/1 -> Add/1

== system tqd/TQD/TorqueDemand/TorqueModule/DriverWhlTqDem/Creep/If Action Subsystem ==
  In1 : Inport
  Action Port : ActionPort
  Out1 : Outport
  wires:
  In1/1 -> Out1/1
